simulink model "controlSystem_TorqueOptimization"  (R2021a)
settings: Solver=VariableStepAuto  StartTime=0.0  StopTime=10.0  RelTol=1e-3
undefined symbols (not defined in the file): brake_constant, however_many_axels_the_brake_is_in_contact_with, mass_of_car, maxEngineTemp, MaxEngineTorque, maxMotorTemp, maxMotorTorque, MaxMotorTorque, radius_of_wheel, sigbuilder_block
libraries: autolibmappedmotor x2, autolibdatasheetbattery x1, autolibsharedmappedengines x1
(part 2 of 2)

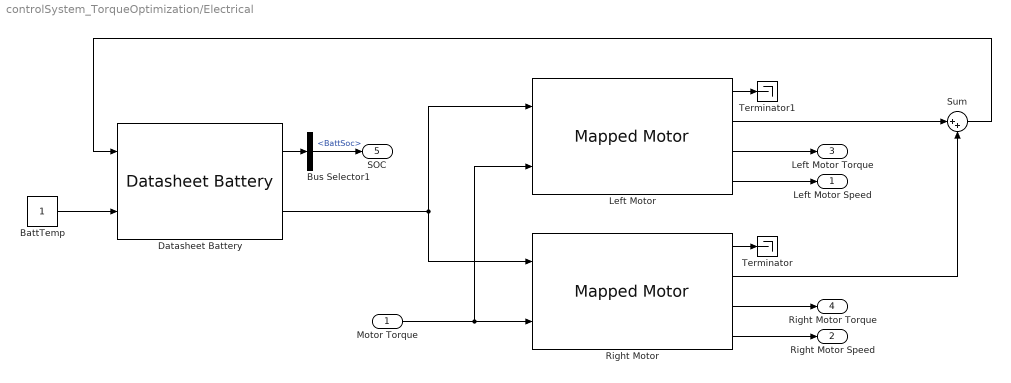
== system controlSystem_TorqueOptimization/Electrical ==
  Motor Torque : Inport
  " Right Motor" : autolibmappedmotor/Mapped Motor  port_config=Torque  param_by=Maximum torque and power  w_t=[ 0 375 750 800 ]  T_t=[0.09 0.08 0.07 0]  torque_max=80  power_max=30  Tc=0.02  param_loss=Single efficiency measurement  eff=100  w_eff=375  T_eff=0.08  Piron=0  Pbase=0  w_eff_bp=[-8000 -4000 0 4000 8000]  T_eff_bp=[0 0.03 0.06 0.09]  Temp_eff_bp=[233.15 293.15 373.15]  losses_table=[1.49 1.67 2.21 3.10; 0.42 0.69 1.14 2.03; 0.06 0.24 0.78 1.68; 0.42 0.69 1.14 2.03; 1.49 1.67 2.21 3.10]  losses_table_3d=cat(3,1.05*[1.49 1.67 2.21 3.10; 0.42 0.69 1.14 2.03; 0.06 0.24 0.78 1.68; 0.42 0.69 1.14 2.03; 1.49 1.67 2.21 3.10],[1.49 1.67 2.21 3.10; 0.42 0.69 1.14 2.03; 0.06 0.24 0.78 1.68; 0.42 0.69 1.14 2.03; 1.49 1.67 2.21 3.10],1.03*[1.49 1.67 2.21 3.10; 0.42 0.69 1.14 2.03; 0.06 0.24 0.78 1.68; 0.42 0.69 1.14 2.03; 1.49 1.67 2.21 3.10])  efficiency_table=[95 95 95 95; 95 95 95 95; 95 95 95 95; 95 95 95 95; 95 95 95 95]  efficiency_table_3d=cat(3,90*ones(5,4),95*ones(5,4),92*ones(5,4))  J=5e-6  b=1e-5  omega_o=0  T_t_extended=[0 0.07 0.08 0.09 0.08 0.07 0]  w_t_extended=[-800 -750 -375 0 375 750 800]  KLossIron=0  KLossCopper=0  x_w_eff_vec=[-8000 -4000 0 4000 8000]  x_T_eff_vec=[-0.09 -0.06 -0.03 0 0.03 0.06 0.09]  x_tmp_eff_vec=[233.15 293.15 373.15]  x_losses_mat=[3.1 2.21 1.67 1.49 1.67 2.21 3.1;2.03 1.14 0.69 0.42 0.69 1.14 2.03;1.68 0.78 0.24 0.06 0.24 0.78 1.68;2.03 1.14 0.69 0.42 0.69 1.14 2.03;3.1 2.21 1.67 1.49 1.67 2.21 3.1]  x_losses_mat_3d=cat(3,[3.255 2.3205 1.7535 1.5645 1.7535 2.3205 3.255;2.1315 1.197 0.7245 0.441 0.7245 1.197 2.1315;1.764 0.819 0.252 0.063 0.252 0.819 1.764;2.1315 1.197 0.7245 0.441 0.7245 1.197 2.1315;3.255 2.3205 1.7535 1.5645 1.7535 2.3205 3.255],[3.1 2.21 1.67 1.49 1.67 2.21 3.1;2.03 1.14 0.69 0.42 0.69 1.14 2.03;1.68 0.78 0.24 0.06 0.24 0.78 1.68;2.03 1.14 0.69 0.42 0.69 1.14 2.03;3.1 2.21 1.67 1.49 1.67 2.21 3.1],[3.193 2.2763 1.7201 1.5347 1.7201 2.2763 3.193;2.0909 1.1742 0.7107 0.4326 0.7107 1.1742 2.0909;1.7304 0.8034 0.2472 0.0618 0.2472 0.8034 1.7304;2.0909 1.1742 0.7107 0.4326 0.7107 1.1742 2.0909;3.193 2.2763 1.7201 1.5347 1.7201 2.2763 3.193])  CalLossMapData={}  CalLossWithTempMapData={}  aMode=2  RefBlkName='autolibmappedmotor/Mapped Motor'
      settings: SourceProductBaseCode=PW,DR,MT,UV,VE
  BattTemp : Constant
  Bus Selector1 : BusSelector  OutputSignals=BattSoc
  Datasheet Battery : autolibdatasheetbattery/Datasheet Battery  CapacityCtrl=Parameter  OutputVlt=Unfiltered  BattChargeMax=100  Em=[2.8 3.228 3.284 3.361 3.408 3.427 3.472 3.477 3.493 3.504 3.516 3.528 3.537 3.545 3.555 3.561 3.566 3.576 3.587 3.589 3.594 3.6 3.608 3.61 3.616 3.619 3.626 3.632 3.637 3.64 3.645 3.646 3.652 3.655 3.658 3.661 3.664 3.668 3.673 3.678 3.68 3.681 3.686 3.692 3.699 3.702 3.705 3.71 3.717 3.723 3.728 3.733 3.735 3.742 3.749 3.755 3.761 3.768 3.773 3.78 3.791 3.798 3.798 3.814 3.818 3.825 3.841 3.846 3.855 3.863 3.877 3.885 3.894 3.907 3.919 3.926 3.935 3.944 3.954 3.964 3.974 3.988 3.998 4.014 4.029 4.034 4.047 4.065 4.074 4.086 4.097 4.131 4.126 4.138 4.15 4.18 4.174 4.187 4.207 4.231 4.221]  CapLUTBp=[0 0.01 0.02 0.03 0.04 0.05 0.06 0.07 0.08 0.09 0.1 0.11 0.12 0.13 0.14 0.15 0.16 0.17 0.18 0.19 0.2 0.21 0.22 0.23 0.24 0.25 0.26 0.27 0.28 0.29 0.3 0.31 0.32 0.33 0.34 0.35 0.36 0.37 0.38 0.39 0.4 0.41 0.42 0.43 0.44 0.45 0.46 0.47 0.48 0.49 0.5 0.51 0.52 0.53 0.54 0.55 0.56 0.57 0.58 0.59 0.6 0.61 0.62 0.63 0.64 0.65 0.66 0.67 0.68 0.69 0.7 0.71 0.72 0.73 0.74 0.75 0.76 0.77 0.78 0.79 0.8 0.81 0.82 0.83 0.84 0.85 0.86 0.87 0.88 0.89 0.9 0.91 0.92 0.93 0.94 0.95 0.96 0.97 0.98 0.99 1]  RInt=[0.008846 0.009319 0.009027 0.00847 0.01032 0.01314;0.006389 0.006554 0.005553 0.005525 0.006043 0.007805;0.004364 0.004101 0.00406 0.003452 0.003846 0.004517;0.002031 0.002563 0.002532 0.00246 0.002716 0.003047;0.001443 0.001825 0.001795 0.001778 0.001924 0.002234;0.0005603 0.0007192 0.0006887 0.0007557 0.0007355 0.001014;0.001028 0.001338 0.001 0.001536 0.001546 0.002789]  BattTempBp=[243.1 253.1 263.1 273.1 283.1 298.1 313.1]  CapSOCBp=[0 0.2 0.4 0.6 0.8 1]  Ns=28  Np=18  BattCapInit=100  Tc=1/1000  Vinit=4.221  RefBlkName='autolibdatasheetbattery/Datasheet Battery'
      settings: SourceProductBaseCode=PW
  Left Motor : autolibmappedmotor/Mapped Motor  port_config=Torque  param_by=Maximum torque and power  w_t=[ 0 375 750 800 ]  T_t=[0.09 0.08 0.07 0]  torque_max=80  power_max=30  Tc=0.02  param_loss=Single efficiency measurement  eff=100  w_eff=375  T_eff=0.08  Piron=0  Pbase=0  w_eff_bp=[-8000 -4000 0 4000 8000]  T_eff_bp=[0 0.03 0.06 0.09]  Temp_eff_bp=[233.15 293.15 373.15]  losses_table=[1.49 1.67 2.21 3.10; 0.42 0.69 1.14 2.03; 0.06 0.24 0.78 1.68; 0.42 0.69 1.14 2.03; 1.49 1.67 2.21 3.10]  losses_table_3d=cat(3,1.05*[1.49 1.67 2.21 3.10; 0.42 0.69 1.14 2.03; 0.06 0.24 0.78 1.68; 0.42 0.69 1.14 2.03; 1.49 1.67 2.21 3.10],[1.49 1.67 2.21 3.10; 0.42 0.69 1.14 2.03; 0.06 0.24 0.78 1.68; 0.42 0.69 1.14 2.03; 1.49 1.67 2.21 3.10],1.03*[1.49 1.67 2.21 3.10; 0.42 0.69 1.14 2.03; 0.06 0.24 0.78 1.68; 0.42 0.69 1.14 2.03; 1.49 1.67 2.21 3.10])  efficiency_table=[95 95 95 95; 95 95 95 95; 95 95 95 95; 95 95 95 95; 95 95 95 95]  efficiency_table_3d=cat(3,90*ones(5,4),95*ones(5,4),92*ones(5,4))  J=5e-6  b=1e-5  omega_o=0  T_t_extended=[0 0.07 0.08 0.09 0.08 0.07 0]  w_t_extended=[-800 -750 -375 0 375 750 800]  KLossIron=0  KLossCopper=0  x_w_eff_vec=[-8000 -4000 0 4000 8000]  x_T_eff_vec=[-0.09 -0.06 -0.03 0 0.03 0.06 0.09]  x_tmp_eff_vec=[233.15 293.15 373.15]  x_losses_mat=[3.1 2.21 1.67 1.49 1.67 2.21 3.1;2.03 1.14 0.69 0.42 0.69 1.14 2.03;1.68 0.78 0.24 0.06 0.24 0.78 1.68;2.03 1.14 0.69 0.42 0.69 1.14 2.03;3.1 2.21 1.67 1.49 1.67 2.21 3.1]  x_losses_mat_3d=cat(3,[3.255 2.3205 1.7535 1.5645 1.7535 2.3205 3.255;2.1315 1.197 0.7245 0.441 0.7245 1.197 2.1315;1.764 0.819 0.252 0.063 0.252 0.819 1.764;2.1315 1.197 0.7245 0.441 0.7245 1.197 2.1315;3.255 2.3205 1.7535 1.5645 1.7535 2.3205 3.255],[3.1 2.21 1.67 1.49 1.67 2.21 3.1;2.03 1.14 0.69 0.42 0.69 1.14 2.03;1.68 0.78 0.24 0.06 0.24 0.78 1.68;2.03 1.14 0.69 0.42 0.69 1.14 2.03;3.1 2.21 1.67 1.49 1.67 2.21 3.1],[3.193 2.2763 1.7201 1.5347 1.7201 2.2763 3.193;2.0909 1.1742 0.7107 0.4326 0.7107 1.1742 2.0909;1.7304 0.8034 0.2472 0.0618 0.2472 0.8034 1.7304;2.0909 1.1742 0.7107 0.4326 0.7107 1.1742 2.0909;3.193 2.2763 1.7201 1.5347 1.7201 2.2763 3.193])  CalLossMapData={}  CalLossWithTempMapData={}  aMode=2  RefBlkName='autolibmappedmotor/Mapped Motor'
      settings: SourceProductBaseCode=PW,DR,MT,UV,VE
  Sum : Sum  Inputs=|++
  Terminator : Terminator
  Terminator1 : Terminator
  Left Motor Speed : Outport
  Right Motor Speed : Outport  Port=2
  Left Motor Torque : Outport  Port=3
  Right Motor Torque : Outport  Port=4
  SOC : Outport  Port=5
  wires:
  BattTemp/1 -> Datasheet Battery/2
  Datasheet Battery/1 -> Bus Selector1/1
  Left Motor/2 -> Sum/1
  " Right Motor"/4 -> Right Motor Speed/1
  Datasheet Battery/2 -> " Right Motor"/1, Left Motor/1
  Left Motor/4 -> Left Motor Speed/1
  " Right Motor"/2 -> Sum/2
  Left Motor/3 -> Left Motor Torque/1
  " Right Motor"/3 -> Right Motor Torque/1
  Bus Selector1/1 -> SOC/1  "<BattSoc>"
  " Right Motor"/1 -> Terminator/1
  Left Motor/1 -> Terminator1/1
  Motor Torque/1 -> Left Motor/2, " Right Motor"/2
  Sum/1 -> Datasheet Battery/1

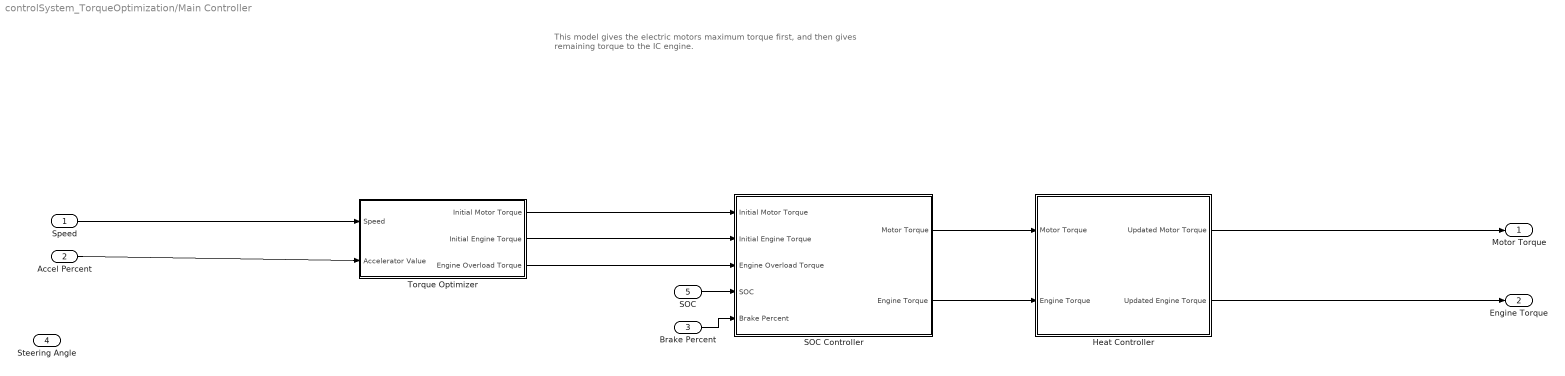
== system controlSystem_TorqueOptimization/Main Controller ==
  note: This model gives the electric motors maximum torque first, and then gives remaining torque to the IC engine.
  Speed : Inport
  Accel Percent : Inport  Port=2
  Brake Percent : Inport  Port=3
  Steering Angle : Inport  Port=4
  SOC : Inport  Port=5
  Heat Controller : Subsystem
  SOC Controller : Subsystem
  Torque Optimizer : Subsystem
  Motor Torque : Outport
  Engine Torque : Outport  Port=2
  wires:
  SOC Controller/1(Motor Torque) -> Heat Controller/1(Motor Torque)
  SOC/1 -> SOC Controller/4(SOC)
  Heat Controller/1(Updated Motor Torque) -> Motor Torque/1
  Heat Controller/2(Updated Engine Torque) -> Engine Torque/1
  SOC Controller/2(Engine Torque) -> Heat Controller/2(Engine Torque)
  Brake Percent/1 -> SOC Controller/5(Brake Percent)
  Accel Percent/1 -> Torque Optimizer/2(Accelerator Value)
  Torque Optimizer/1(Initial Motor Torque) -> SOC Controller/1(Initial Motor Torque)
  Torque Optimizer/2(Initial Engine Torque) -> SOC Controller/2(Initial Engine Torque)
  Torque Optimizer/3(Engine Overload Torque) -> SOC Controller/3(Engine Overload Torque)
  Speed/1 -> Torque Optimizer/1(Speed)

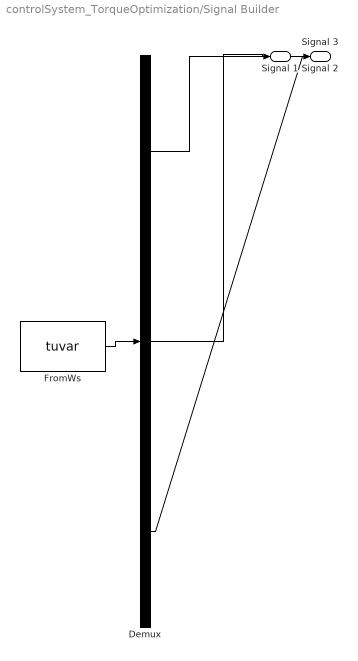
== system controlSystem_TorqueOptimization/Signal Builder ==
  Demux : Demux  Tag=STV Demux  Outputs=3
      settings: DisplayOption=none
  FromWs : FromWorkspace  Tag=STV FromWs  VariableName=tuvar
      SigBuilderData=|
      | common.afterFinalStr = 'Extrapolate'
      | common.sampleTime = 0
      | dataSet.timeRange = [0 10]
      | dataSet.name = 'Group 1'
      | sbobj.Groups.Name = 'Group 1'
      | sbobj.Groups.Signals(1).Name = 'Signal 1'
      | sbobj.Groups.Signals(1).XData = [0 5 5 10]
      | sbobj.Groups.Signals(1).YData = [0.1 0.94 0.06 0.06]
      | sbobj.Groups.Signals(2).Name = 'Signal 2'
      | sbobj.Groups.Signals(2).XData = [0 5 5 10]
      | sbobj.Groups.Signals(2).YData = [0 0 0.02 1]
      | sbobj.Groups.Signals(3).Name = 'Signal 3'
      | sbobj.Groups.Signals(3).XData = [0 0.25 0.5 0.75 1 1.25 1.5 1.75 2 2.25 2.5 2.75 3 3.25 3.5 3.75 4 4.25 4.5 4.75 5 5.25 5.5 5.75 6 6.25 6.5 6.75 7 7.25 7.5 7.75 8 8.25 8.5 8.75 9 9.25 9.5 9.75 10]
      | sbobj.Groups.Signals(3).YData = [0 3.53553390593 5 3.53553390593 6.12323399574e-16 -3.53553390593 -5 -3.53553390593 0 3.53553390593 5 3.53553390593 6.12323399574e-16 -3.53553390593 -5 -3.53553390593 0 3.53553390593 5 3.53553390593 6.12323399574e-16 -3.53553390593 -5 -3.53553390593 0 3.53553390593 5 3.53553390593 6.12323399574e-16 -3.53553390593 -5 -3.53553390593 0 3.53553390593 5 3.53553390593 6.12323399574e-16 -3.53553390593 -5 -3.53553390593 0]
  Signal 1 : Outport  Tag=STV Outport
  Signal 2 : Outport  Tag=STV Outport  Port=2
  Signal 3 : Outport  Tag=STV Outport  Port=3
  wires:
  Demux/1 -> Signal 1/1
  FromWs/1 -> Demux/1
  Demux/2 -> Signal 2/1
  Demux/3 -> Signal 3/1

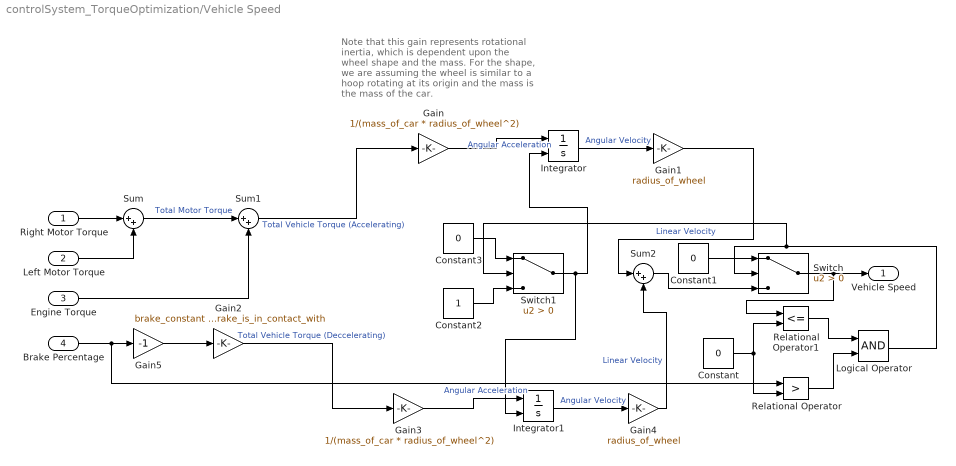
== system controlSystem_TorqueOptimization/Vehicle Speed ==
  note: Note that this gain represents rotational inertia, which is dependent upon the wheel shape and the mass. For the shape, we are assuming the wheel is similar to a hoop rotating at its origin and the mass is the mass of the car.
  Right Motor Torque : Inport
  Left Motor Torque : Inport  Port=2
  Engine Torque : Inport  Port=3
  Brake Percentage : Inport  Port=4
  Constant : Constant  Value=0
  Constant1 : Constant  Value=0
  Constant2 : Constant
  Constant3 : Constant  Value=0
  Gain : Gain  Gain=1/(mass_of_car * radius_of_wheel^2)
  Gain1 : Gain  Gain=radius_of_wheel
  Gain2 : Gain  Gain=brake_constant * however_many_axels_the_brake_is_in_contact_with
  Gain3 : Gain  Gain=1/(mass_of_car * radius_of_wheel^2)
  Gain4 : Gain  Gain=radius_of_wheel
  Gain5 : Gain  Gain=-1
  Integrator : Integrator  ExternalReset=falling
  Integrator1 : Integrator  ExternalReset=falling
  Logical Operator : Logic  AllPortsSameDT=off  OutDataTypeStr=boolean
  Relational Operator : RelationalOperator  Operator=>  OutDataTypeStr=boolean  RndMeth=Simplest
  Relational Operator1 : RelationalOperator  Operator=<=  OutDataTypeStr=boolean  RndMeth=Simplest
  Sum : Sum  Inputs=|++
  Sum1 : Sum  Inputs=|++
  Sum2 : Sum  Inputs=|++
  Switch : Switch  Criteria=u2 > Threshold
  Switch1 : Switch  Criteria=u2 > Threshold
  Vehicle Speed : Outport
  wires:
  Right Motor Torque/1 -> Sum/1
  Left Motor Torque/1 -> Sum/2
  Engine Torque/1 -> Sum1/2
  Sum/1 -> Sum1/1  "Total Motor Torque"
  Sum1/1 -> Gain/1  "Total Vehicle Torque (Accelerating)"
  Gain/1 -> Integrator/1  "Angular Acceleration"
  Integrator/1 -> Gain1/1  "Angular Velocity"
  Gain1/1 -> Sum2/1  "Linear Velocity"
  Gain3/1 -> Integrator1/1  "Angular Acceleration"
  Integrator1/1 -> Gain4/1  "Angular Velocity"
  Gain2/1 -> Gain3/1  "Total Vehicle Torque (Deccelerating)"
  Gain4/1 -> Sum2/2  "Linear Velocity"
  Sum2/1 -> Switch/3
  Brake Percentage/1 -> Relational Operator/1, Gain5/1
  Gain5/1 -> Gain2/1
  Constant/1 -> Relational Operator/2, Relational Operator1/2
  Relational Operator1/1 -> Logical Operator/1
  Relational Operator/1 -> Logical Operator/2
  Logical Operator/1 -> Switch1/2, Switch/2
  Constant1/1 -> Switch/1
  Switch/1 -> Relational Operator1/1, Vehicle Speed/1
  Switch1/1 -> Integrator1/2, Integrator/2
  Constant3/1 -> Switch1/1
  Constant2/1 -> Switch1/3

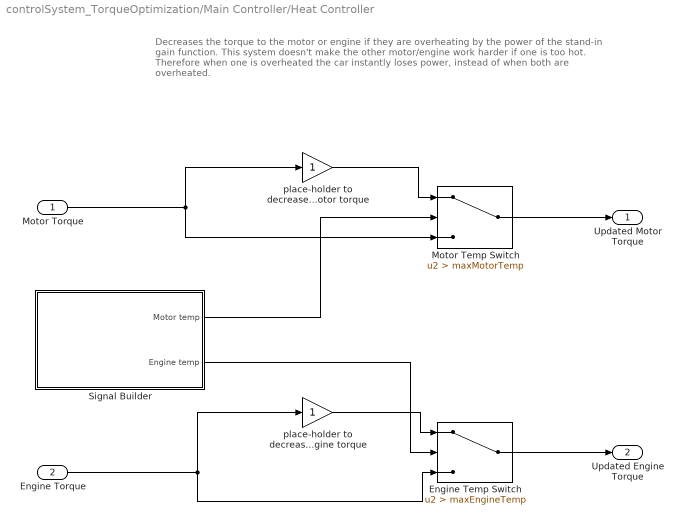
== system controlSystem_TorqueOptimization/Main Controller/Heat Controller ==
  note: Decreases the torque to the motor or engine if they are overheating by the power of the stand-in gain function.
      | This system doesn't make the other motor/engine work harder if one is too hot. Therefore when one is overheated the car instantly loses power, instead of when both are overheated.
  Motor Torque : Inport
  Engine Torque : Inport  Port=2
  Engine Temp Switch : Switch  Criteria=u2 > Threshold  Threshold=maxEngineTemp
  Motor Temp Switch : Switch  Criteria=u2 > Threshold  Threshold=maxMotorTemp
  Signal Builder : Subsystem  Tag=STV Subsys  LoadFcn=sigbuilder_block('load');  StartFcn=sigbuilder_block('start');  StopFcn=sigbuilder_block('stop');  ClipboardFcn=sigbuilder_block('clipboard');  mask(Sigbuilder block){tuvar=[0:10]}
      mask help: Simulink:masks:SigbuilderBlock_MD
      mask init:
      | if ~strcmp(get_param(bdroot(gcbh),'SimulationStatus'),'stopped') tuvar = sigbuilder_block('maskInit'); end
      settings: CopyFcn=sigbuilder_block('copy');  DeleteFcn=sigbuilder_block('delete');  ModelCloseFcn=sigbuilder_block('modelClose');  PreSaveFcn=sigbuilder_block('preSave');  PauseFcn=sigbuilder_block('pause');  ContinueFcn=sigbuilder_block('continue');  NameChangeFcn=sigbuilder_block('namechange');  OpenFcn=sigbuilder_block('open',[411 128.5 543.5 351.5 ]);  CloseFcn=sigbuilder_block('close');
      mask Display: plot(0, 0, 100, 100,[2, 2, 32, 32, 2], [68, 8, 8, 68, 68],[32, 2], [38, 38], [32, 19, 2],[53, 60, 44], [32, 17, 17, 2],[16, 16, 31, 31]);txt = getActiveGroup(gcbh);text(2, 100, txt,'verticalAlignment', 'top');
  place-holder to decrease engine torque : Gain
  place-holder to decrease motor torque : Gain
  Updated Motor Torque : Outport
  Updated Engine Torque : Outport  Port=2
  wires:
  Motor Torque/1 -> place-holder to decrease motor torque/1, Motor Temp Switch/3
  place-holder to decrease motor torque/1 -> Motor Temp Switch/1
  Engine Torque/1 -> place-holder to decrease engine torque/1, Engine Temp Switch/3
  place-holder to decrease engine torque/1 -> Engine Temp Switch/1
  Signal Builder/1(Motor temp) -> Motor Temp Switch/2
  Signal Builder/2(Engine temp) -> Engine Temp Switch/2
  Motor Temp Switch/1 -> Updated Motor Torque/1
  Engine Temp Switch/1 -> Updated Engine Torque/1

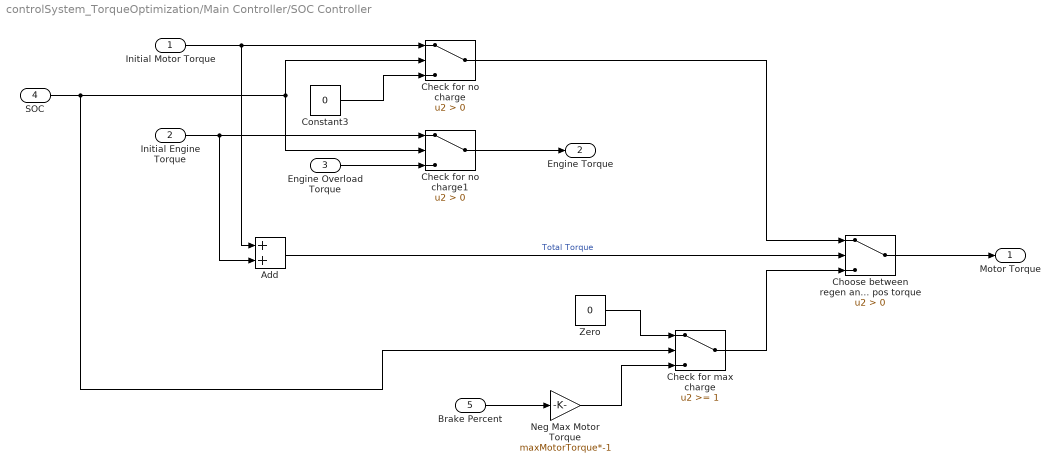
== system controlSystem_TorqueOptimization/Main Controller/SOC Controller ==
  Initial Motor Torque : Inport
  Initial Engine Torque : Inport  Port=2
  Engine Overload Torque : Inport  Port=3
  SOC : Inport  Port=4
  Brake Percent : Inport  Port=5
  Add : Sum
  Check for max charge : Switch  Threshold=1
  Check for no charge : Switch  Criteria=u2 > Threshold
  Check for no charge1 : Switch  Criteria=u2 > Threshold
  Choose between regen and pos torque : Switch  Criteria=u2 > Threshold
  Constant3 : Constant  Value=0
  Neg Max Motor Torque : Gain  Gain=maxMotorTorque*-1
  Zero : Constant  Value=0  OutDataTypeStr=Inherit: Inherit via back propagation
  Motor Torque : Outport
  Engine Torque : Outport  Port=2
  wires:
  Check for no charge1/1 -> Engine Torque/1
  Engine Overload Torque/1 -> Check for no charge1/3
  Constant3/1 -> Check for no charge/3
  Check for no charge/1 -> Choose between regen and pos torque/1
  Initial Motor Torque/1 -> Add/1, Check for no charge/1
  Initial Engine Torque/1 -> Add/2, Check for no charge1/1
  Brake Percent/1 -> Neg Max Motor Torque/1
  Add/1 -> Choose between regen and pos torque/2  "Total Torque"
  Choose between regen and pos torque/1 -> Motor Torque/1
  SOC/1 -> Check for no charge1/2, Check for no charge/2, Check for max charge/2
  Zero/1 -> Check for max charge/1
  Neg Max Motor Torque/1 -> Check for max charge/3
  Check for max charge/1 -> Choose between regen and pos torque/3

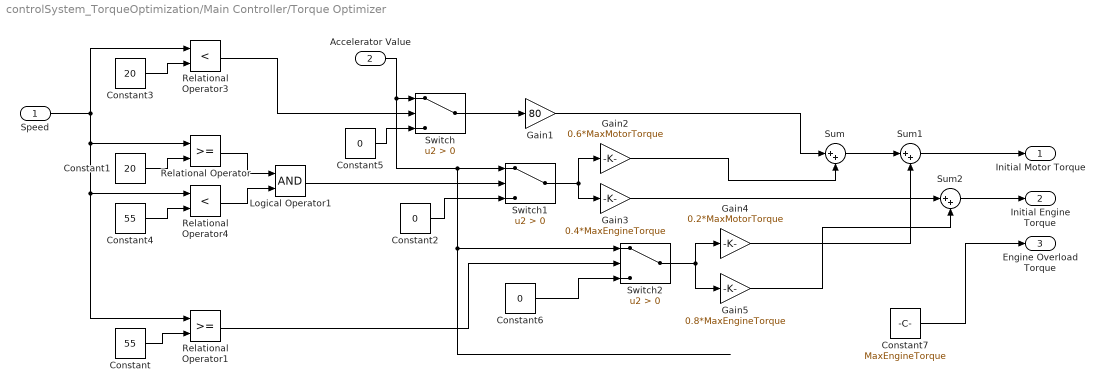
== system controlSystem_TorqueOptimization/Main Controller/Torque Optimizer ==
  Speed : Inport
  Accelerator Value : Inport  Port=2
  Constant : Constant  Value=55
  Constant1 : Constant  Value=20
  Constant2 : Constant  Value=0
  Constant3 : Constant  Value=20
  Constant4 : Constant  Value=55
  Constant5 : Constant  Value=0
  Constant6 : Constant  Value=0
  Constant7 : Constant  Value=MaxEngineTorque
  Gain1 : Gain  Gain=80
  Gain2 : Gain  Gain=0.6*MaxMotorTorque
  Gain3 : Gain  Gain=0.4*MaxEngineTorque
  Gain4 : Gain  Gain=0.2*MaxMotorTorque
  Gain5 : Gain  Gain=0.8*MaxEngineTorque
  Logical Operator1 : Logic  AllPortsSameDT=off  OutDataTypeStr=boolean
  Relational Operator : RelationalOperator  OutDataTypeStr=boolean  RndMeth=Simplest
  Relational Operator1 : RelationalOperator  OutDataTypeStr=boolean  RndMeth=Simplest
  Relational Operator3 : RelationalOperator  Operator=<  OutDataTypeStr=boolean  RndMeth=Simplest
  Relational Operator4 : RelationalOperator  Operator=<  OutDataTypeStr=boolean  RndMeth=Simplest
  Sum : Sum  Inputs=|++
  Sum1 : Sum  Inputs=|++
  Sum2 : Sum  Inputs=|++
  Switch : Switch  Criteria=u2 > Threshold
  Switch1 : Switch  Criteria=u2 > Threshold
  Switch2 : Switch  Criteria=u2 > Threshold
  Initial Motor Torque : Outport
  Initial Engine Torque : Outport  Port=2
  Engine Overload Torque : Outport  Port=3
  wires:
  Constant1/1 -> Relational Operator/2
  Constant/1 -> Relational Operator1/2
  Constant3/1 -> Relational Operator3/2
  Constant4/1 -> Relational Operator4/2
  Relational Operator/1 -> Logical Operator1/1
  Relational Operator4/1 -> Logical Operator1/2
  Speed/1 -> Relational Operator/1, Relational Operator1/1, Relational Operator4/1, Relational Operator3/1
  Relational Operator1/1 -> Switch2/2
  Logical Operator1/1 -> Switch1/2
  Relational Operator3/1 -> Switch/2
  Accelerator Value/1 -> Switch2/1, Switch1/1, Switch/1
  Sum/1 -> Sum1/1
  Constant5/1 -> Switch/3
  Constant2/1 -> Switch1/3
  Constant6/1 -> Switch2/3
  Switch2/1 -> Gain5/1, Gain4/1
  Switch1/1 -> Gain3/1, Gain2/1
  Switch/1 -> Gain1/1
  Gain1/1 -> Sum/1
  Gain2/1 -> Sum/2
  Gain4/1 -> Sum1/2
  Sum1/1 -> Initial Motor Torque/1
  Sum2/1 -> Initial Engine Torque/1
  Gain3/1 -> Sum2/1
  Gain5/1 -> Sum2/2
  Constant7/1 -> Engine Overload Torque/1

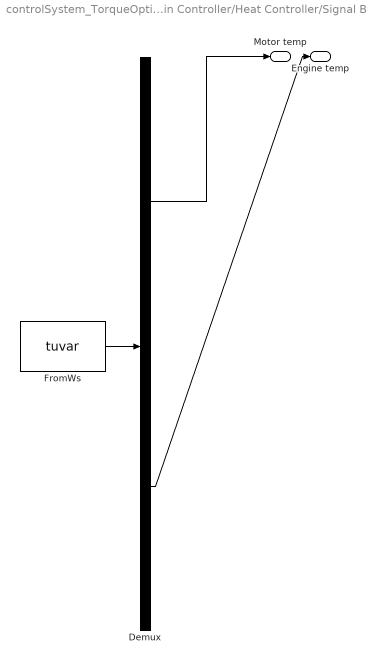
== system controlSystem_TorqueOptimization/Main Controller/Heat Controller/Signal Builder ==
  Demux : Demux  Tag=STV Demux  Outputs=2
      settings: DisplayOption=none
  FromWs : FromWorkspace  Tag=STV FromWs  VariableName=tuvar
      SigBuilderData=|
      | common.afterFinalStr = 'Extrapolate'
      | common.sampleTime = 0
      | dataSet.timeRange = [0 10]
      | dataSet.name = 'Temperature Signals'
      | sbobj.Groups.Name = 'Temperature Signals'
      | sbobj.Groups.Signals(1).Name = 'Motor temp'
      | sbobj.Groups.Signals(1).XData = [0 10]
      | sbobj.Groups.Signals(1).YData = [0 0]
      | sbobj.Groups.Signals(2).Name = 'Engine temp'
      | sbobj.Groups.Signals(2).XData = [0 10]
      | sbobj.Groups.Signals(2).YData = [0 0]
  Motor temp : Outport  Tag=STV Outport
  Engine temp : Outport  Tag=STV Outport  Port=2
  wires:
  FromWs/1 -> Demux/1
  Demux/1 -> Motor temp/1
  Demux/2 -> Engine temp/1
